simulink model "working"  (R2018b)
settings: Solver=FixedStepDiscrete  StartTime=0.0  StopTime=20  FixedStep=Ts  RelTol=1e-3
undefined symbols (not defined in the file): b, DiscIntNeverNeededParam, g, I, l, m, M, Ts
libraries: fuzblock x2
settings Model: Creator=Kamran  LastModifiedBy=Sepid

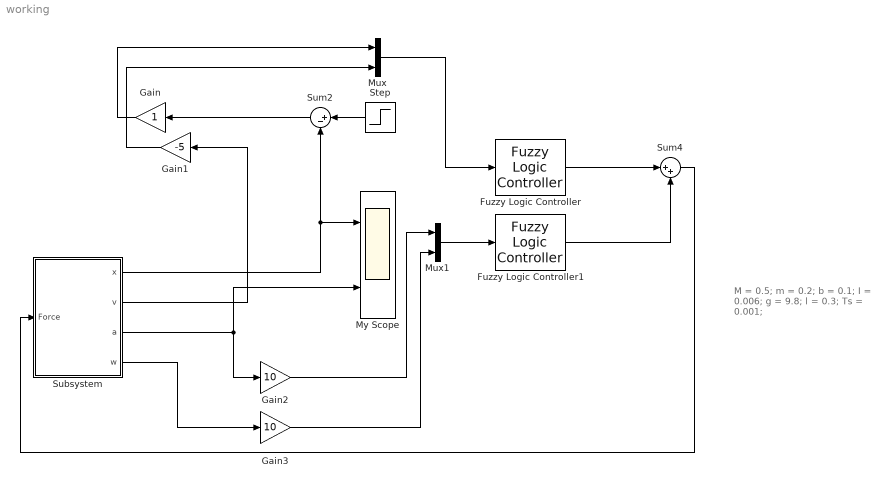
== system working ==
  note: M = 0.5;
      | m = 0.2;
      | b = 0.1;
      | I = 0.006;
      | g = 9.8;
      | l = 0.3;
      | Ts = 0.001;
  Fuzzy Logic Controller : fuzblock/Fuzzy Logic  Controller  FIS='x'  OutputSampleNumber=101  DataType=double  FuzzifiedInputs=off  RuleFiringStrengths=off  RuleOutputs=off  AggregatedOutputs=off  SimulateUsing=Interpreted execution  OutOfRangeInputValueMessage=warning  NoRuleFiredMessage=warning  EmptyOutputFuzzySetMessage=warning
  Fuzzy Logic Controller1 : fuzblock/Fuzzy Logic  Controller  FIS='theta'  OutputSampleNumber=101  DataType=double  FuzzifiedInputs=off  RuleFiringStrengths=off  RuleOutputs=off  AggregatedOutputs=off  SimulateUsing=Interpreted execution  OutOfRangeInputValueMessage=warning  NoRuleFiredMessage=warning  EmptyOutputFuzzySetMessage=warning
  Gain : Gain
  Gain1 : Gain  Gain=-5
  Gain2 : Gain  Gain=10
  Gain3 : Gain  Gain=10
  Mux : Mux  Inputs=2
  Mux1 : Mux  Inputs=2
  My Scope : Scope  NumInputPorts=2
  Step : Step  After=0  SampleTime=Ts
  Subsystem : Subsystem  mask{X0=5, A0=0.18}
      mask prompts: X0 "Initial Pos"; A0 "Initial Angle"
  Sum2 : Sum  Inputs=|+-
  Sum4 : Sum  Inputs=|++
  wires:
  Subsystem/3(a) -> Gain2/1, My Scope/2
  Subsystem/1(x) -> Sum2/2, My Scope/1
  Step/1 -> Sum2/1
  Sum2/1 -> Gain/1
  Mux/1 -> Fuzzy Logic Controller/1
  Mux1/1 -> Fuzzy Logic Controller1/1
  Fuzzy Logic Controller/1 -> Sum4/1
  Fuzzy Logic Controller1/1 -> Sum4/2
  Sum4/1 -> Subsystem/1(Force)
  Gain3/1 -> Mux1/2
  Gain2/1 -> Mux1/1
  Gain1/1 -> Mux/2
  Gain/1 -> Mux/1
  Subsystem/4(w) -> Gain3/1
  Subsystem/2(v) -> Gain1/1

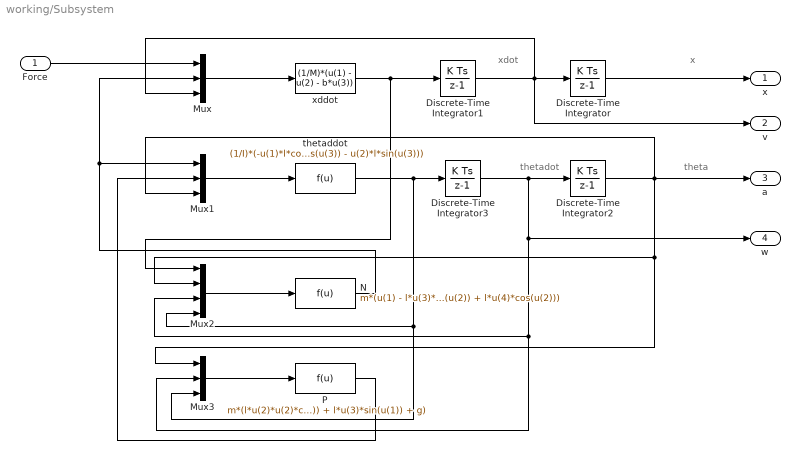
== system working/Subsystem ==
  note: theta
  note: x
  note: thetadot
  note: xdot
  Force : Inport
  Discrete-Time Integrator : DiscreteIntegrator  InitialCondition=X0  SampleTime=-1  ICPrevOutput=DiscIntNeverNeededParam  ICPrevScaledInput=DiscIntNeverNeededParam
  Discrete-Time Integrator1 : DiscreteIntegrator  SampleTime=-1  ICPrevOutput=DiscIntNeverNeededParam  ICPrevScaledInput=DiscIntNeverNeededParam
  Discrete-Time Integrator2 : DiscreteIntegrator  InitialCondition=A0  SampleTime=-1  ICPrevOutput=DiscIntNeverNeededParam  ICPrevScaledInput=DiscIntNeverNeededParam
  Discrete-Time Integrator3 : DiscreteIntegrator  SampleTime=-1  ICPrevOutput=DiscIntNeverNeededParam  ICPrevScaledInput=DiscIntNeverNeededParam
  Mux : Mux  Inputs=3
  Mux1 : Mux  Inputs=3
  Mux2 : Mux
  Mux3 : Mux  Inputs=3
  N : Fcn  Expr=m*(u(1) - l*u(3)*u(3)*sin(u(2)) + l*u(4)*cos(u(2)))
  P : Fcn  Expr=m*(l*u(2)*u(2)*cos(u(1)) + l*u(3)*sin(u(1)) + g)
  thetaddot : Fcn  Expr=(1/I)*(-u(1)*l*cos(u(3)) - u(2)*l*sin(u(3)))
  xddot : Fcn  Expr=(1/M)*(u(1) - u(2) - b*u(3))
  x : Outport
  v : Outport  Port=2
  a : Outport  Port=3
  w : Outport  Port=4
  wires:
  Force/1 -> Mux/1
  Mux2/1 -> N/1
  Mux/1 -> xddot/1
  P/1 -> Mux1/2
  Mux3/1 -> P/1
  N/1 -> Mux1/1, Mux/2
  Mux1/1 -> thetaddot/1
  xddot/1 -> Discrete-Time Integrator1/1, Mux2/1
  Discrete-Time Integrator/1 -> x/1
  thetaddot/1 -> Mux3/3, Mux2/4, Discrete-Time Integrator3/1
  Discrete-Time Integrator1/1 -> v/1, Mux/3, Discrete-Time Integrator/1
  Discrete-Time Integrator3/1 -> Mux2/3, Mux3/2, w/1, Discrete-Time Integrator2/1
  Discrete-Time Integrator2/1 -> Mux3/1, Mux2/2, a/1, Mux1/3
